simulink model "trajec_motion"  (R2016b)
settings: Solver=VariableStepAuto  StartTime=0.0  StopTime=10  RelTol=1e-3
undefined symbols (not defined in the file): X, Y, Z
libraries: sm_lib x12, nesl_utility x9, simulink x6
settings Model: Creator=macbookpro  LastModifiedBy=macbookpro
settings SimscapeCC: SimscapeLogType=all  SimscapeLogDataHistory=10000

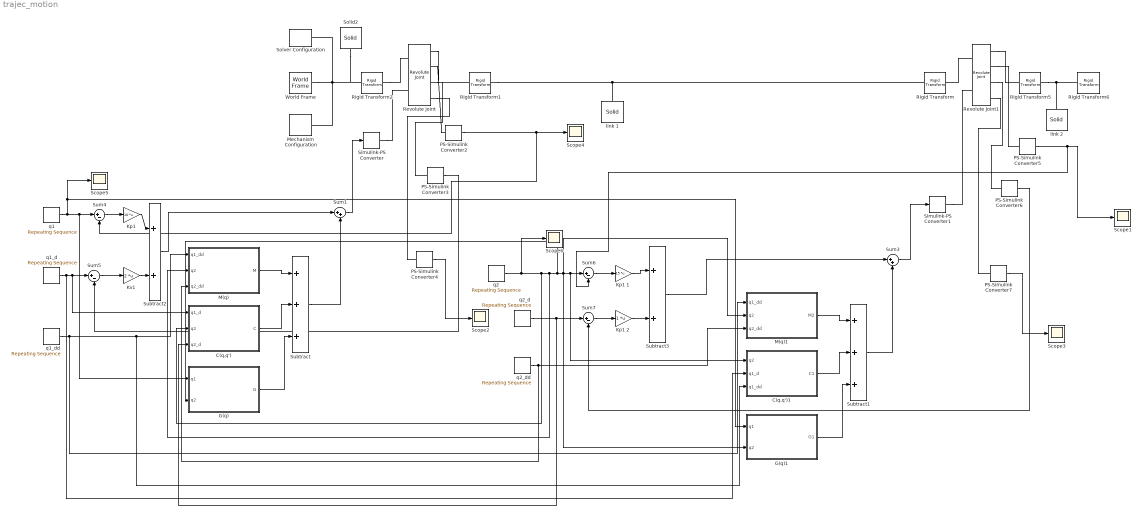
== system trajec_motion ==
  C(q,q') : MATLAB Function  TreatAsAtomicUnit=on
  C(q,q')1 : MATLAB Function  TreatAsAtomicUnit=on
  G(q) : MATLAB Function  TreatAsAtomicUnit=on
  G(q)1 : MATLAB Function  TreatAsAtomicUnit=on
  "Kp1 " : Gain  Gain=10  Multiplication=Matrix(K*u) (u vector)
  Kp1 1 : Gain  Gain=15  Multiplication=Matrix(K*u) (u vector)
  Kp1 2 : Gain  Multiplication=Matrix(K*u) (u vector)
  Kv1 : Gain  Gain=2  Multiplication=Matrix(K*u) (u vector)
  M(q) : MATLAB Function  TreatAsAtomicUnit=on
  M(q)1 : MATLAB Function  TreatAsAtomicUnit=on
  Mechanism Configuration : sm_lib/Utilities/Mechanism Configuration  UniformGravity=Constant  GravityVector=[0 0 -9.80665]  GravityUnits=m/s^2  LinearizationDelta=0.001
  PS-Simulink Converter2 : nesl_utility/PS-Simulink Converter  PhysicalDomain=network_engine_domain  SubClassName=ps_output  LeftPortType=input  RightPortType=output  PseudoPeriodic=off  Frequencies=[]  Unit=rad  AffineConversion=off
  PS-Simulink Converter3 : nesl_utility/PS-Simulink Converter  PhysicalDomain=network_engine_domain  SubClassName=ps_output  LeftPortType=input  RightPortType=output  PseudoPeriodic=off  Frequencies=[]  Unit=rad/s  AffineConversion=off
  PS-Simulink Converter4 : nesl_utility/PS-Simulink Converter  PhysicalDomain=network_engine_domain  SubClassName=ps_output  LeftPortType=input  RightPortType=output  PseudoPeriodic=off  Frequencies=[]  Unit=1  AffineConversion=off
  PS-Simulink Converter5 : nesl_utility/PS-Simulink Converter  PhysicalDomain=network_engine_domain  SubClassName=ps_output  LeftPortType=input  RightPortType=output  PseudoPeriodic=off  Frequencies=[]  Unit=rad  AffineConversion=off
  PS-Simulink Converter6 : nesl_utility/PS-Simulink Converter  PhysicalDomain=network_engine_domain  SubClassName=ps_output  LeftPortType=input  RightPortType=output  PseudoPeriodic=off  Frequencies=[]  Unit=rad/s  AffineConversion=off
  PS-Simulink Converter7 : nesl_utility/PS-Simulink Converter  PhysicalDomain=network_engine_domain  SubClassName=ps_output  LeftPortType=input  RightPortType=output  PseudoPeriodic=off  Frequencies=[]  Unit=1  AffineConversion=off
  Revolute Joint : sm_lib/Joints/Revolute Joint  SenseConstraintForce=off  SenseConstraintForceX=off  SenseConstraintForceY=off  SenseConstraintForceZ=off  SenseConstraintTorque=off  SenseConstraintTorqueX=off  SenseConstraintTorqueY=off  SenseConstraintTorqueZ=off  SenseTotalForce=off  SenseTotalForceX=off  SenseTotalForceY=off  SenseTotalForceZ=off  SenseTotalTorque=off  SenseTotalTorqueX=off  SenseTotalTorqueY=off  SenseTotalTorqueZ=off  CompositeWrenchDir=FollowerOnBase  CompositeWrenchFrame=BaseFrame  EquilibriumPosition=0  EquilibriumPositionUnits=rad  SpringStiffness=1  SpringStiffnessUnits=N*m/rad  DampingCoefficient=0.01  DampingCoefficientUnits=N*m/(rad/s)  TorqueActuationMode=InputTorque  MotionActuationMode=ComputedMotion  SensePosition=on  SenseVelocity=on  SenseAcceleration=on  SenseTorqueForce=off  PositionTargetSpecify=off  PositionTargetPriority=High  PositionTargetValue=30  PositionTargetValueUnits=deg  VelocityTargetSpecify=off  VelocityTargetPriority=High  VelocityTargetValue=0  VelocityTargetValueUnits=deg/s
  Revolute Joint1 : sm_lib/Joints/Revolute Joint  SenseConstraintForce=off  SenseConstraintForceX=off  SenseConstraintForceY=off  SenseConstraintForceZ=off  SenseConstraintTorque=off  SenseConstraintTorqueX=off  SenseConstraintTorqueY=off  SenseConstraintTorqueZ=off  SenseTotalForce=off  SenseTotalForceX=off  SenseTotalForceY=off  SenseTotalForceZ=off  SenseTotalTorque=off  SenseTotalTorqueX=off  SenseTotalTorqueY=off  SenseTotalTorqueZ=off  CompositeWrenchDir=FollowerOnBase  CompositeWrenchFrame=BaseFrame  EquilibriumPosition=0  EquilibriumPositionUnits=rad  SpringStiffness=1  SpringStiffnessUnits=N*m/rad  DampingCoefficient=0.01  DampingCoefficientUnits=N*m/(rad/s)  TorqueActuationMode=InputTorque  MotionActuationMode=ComputedMotion  SensePosition=on  SenseVelocity=on  SenseAcceleration=on  SenseTorqueForce=off  PositionTargetSpecify=off  PositionTargetPriority=High  PositionTargetValue=30  PositionTargetValueUnits=deg  VelocityTargetSpecify=off  VelocityTargetPriority=High  VelocityTargetValue=0  VelocityTargetValueUnits=deg/s
  Rigid Transform : sm_lib/Frames and Transforms/Rigid Transform  TranslationMethod=StandardAxis  TranslationStandardOffset=0.41/2  TranslationLengthUnit=m  TranslationStandardAxis=+Z  TranslationCartesianOffset=[0 0 0]  TranslationROffset=0  TranslationROffsetUnits=m  TranslationZOffset=0  TranslationZOffsetUnits=m  TranslationThetaOffset=0  TranslationThetaOffsetUnits=deg  RotationMethod=StandardAxis  RotationAngleUnits=deg  RotationStandardAxis=+X  RotationAngle=90  RotationArbitraryAxis=[0 0 1]  FollAlignAxisA=+X  BaseAlignAxisA=+Y  FollAlignAxisB=+Y  BaseAlignAxisB=+Z  RotationSequenceAxes=FollowerAxes  RotationSequence=XYX  RotationSequenceAngles=[0 0 0]  RotationSequenceAnglesUnits=deg  RotationMatrix=[1 0 0; 0 1 0; 0 0 1]
  Rigid Transform1 : sm_lib/Frames and Transforms/Rigid Transform  TranslationMethod=StandardAxis  TranslationStandardOffset=0.41/2  TranslationLengthUnit=m  TranslationStandardAxis=-Z  TranslationCartesianOffset=[0 0 0]  TranslationROffset=0  TranslationROffsetUnits=m  TranslationZOffset=0  TranslationZOffsetUnits=m  TranslationThetaOffset=0  TranslationThetaOffsetUnits=deg  RotationMethod=StandardAxis  RotationAngleUnits=deg  RotationStandardAxis=+X  RotationAngle=90  RotationArbitraryAxis=[0 0 1]  FollAlignAxisA=+X  BaseAlignAxisA=+Y  FollAlignAxisB=+Y  BaseAlignAxisB=+Z  RotationSequenceAxes=FollowerAxes  RotationSequence=XYX  RotationSequenceAngles=[0 0 0]  RotationSequenceAnglesUnits=deg  RotationMatrix=[1 0 0; 0 1 0; 0 0 1]
  Rigid Transform2 : sm_lib/Frames and Transforms/Rigid Transform  TranslationMethod=None  TranslationStandardOffset=0.41/2  TranslationLengthUnit=m  TranslationStandardAxis=+Z  TranslationCartesianOffset=[0 0 0]  TranslationROffset=0  TranslationROffsetUnits=m  TranslationZOffset=0  TranslationZOffsetUnits=m  TranslationThetaOffset=0  TranslationThetaOffsetUnits=deg  RotationMethod=StandardAxis  RotationAngleUnits=deg  RotationStandardAxis=+X  RotationAngle=90  RotationArbitraryAxis=[0 0 1]  FollAlignAxisA=+X  BaseAlignAxisA=+Y  FollAlignAxisB=+Y  BaseAlignAxisB=+Z  RotationSequenceAxes=FollowerAxes  RotationSequence=XYX  RotationSequenceAngles=[0 0 0]  RotationSequenceAnglesUnits=deg  RotationMatrix=[1 0 0; 0 1 0; 0 0 1]
  Rigid Transform5 : sm_lib/Frames and Transforms/Rigid Transform  TranslationMethod=StandardAxis  TranslationStandardOffset=0.39/2  TranslationLengthUnit=m  TranslationStandardAxis=-Z  TranslationCartesianOffset=[0 0 0]  TranslationROffset=0  TranslationROffsetUnits=m  TranslationZOffset=0  TranslationZOffsetUnits=m  TranslationThetaOffset=0  TranslationThetaOffsetUnits=deg  RotationMethod=StandardAxis  RotationAngleUnits=deg  RotationStandardAxis=+X  RotationAngle=90  RotationArbitraryAxis=[0 0 1]  FollAlignAxisA=+X  BaseAlignAxisA=+Y  FollAlignAxisB=+Y  BaseAlignAxisB=+Z  RotationSequenceAxes=FollowerAxes  RotationSequence=XYX  RotationSequenceAngles=[0 0 0]  RotationSequenceAnglesUnits=deg  RotationMatrix=[1 0 0; 0 1 0; 0 0 1]
  Rigid Transform6 : sm_lib/Frames and Transforms/Rigid Transform  TranslationMethod=StandardAxis  TranslationStandardOffset=0.39/2  TranslationLengthUnit=m  TranslationStandardAxis=+Z  TranslationCartesianOffset=[0 0 0]  TranslationROffset=0  TranslationROffsetUnits=m  TranslationZOffset=0  TranslationZOffsetUnits=m  TranslationThetaOffset=0  TranslationThetaOffsetUnits=deg  RotationMethod=StandardAxis  RotationAngleUnits=deg  RotationStandardAxis=+X  RotationAngle=90  RotationArbitraryAxis=[0 0 1]  FollAlignAxisA=+X  BaseAlignAxisA=+Y  FollAlignAxisB=+Y  BaseAlignAxisB=+Z  RotationSequenceAxes=FollowerAxes  RotationSequence=XYX  RotationSequenceAngles=[0 0 0]  RotationSequenceAnglesUnits=deg  RotationMatrix=[1 0 0; 0 1 0; 0 0 1]
  Scope{1..6} (6 alike) : Scope
  Simulink-PS Converter : nesl_utility/Simulink-PS Converter  PhysicalDomain=network_engine_domain  SubClassName=ps_input  LeftPortType=input  RightPortType=output  PseudoPeriodic=off  Frequencies=[]  NoiseDistribution=none  NoiseParameters=[]  Unit=N*m  AffineConversion=off  InputFiltering=on  SimscapeFilterOrder=2  InputFilterTimeConstant=0.01  UdotUserProvided=1
  Simulink-PS Converter1 : nesl_utility/Simulink-PS Converter  PhysicalDomain=network_engine_domain  SubClassName=ps_input  LeftPortType=input  RightPortType=output  PseudoPeriodic=off  Frequencies=[]  NoiseDistribution=none  NoiseParameters=[]  Unit=N*m  AffineConversion=off  InputFiltering=on  SimscapeFilterOrder=2  InputFilterTimeConstant=0.01  UdotUserProvided=1
  Solid2 : sm_lib/Body Elements/Solid  InertiaType=CalculateFromGeometry  Mass=1  MassUnits=kg  CenterOfMass=[0 0 0]  CenterOfMassUnits=m  MomentsOfInertia=[1 1 1]  MomentsOfInertiaUnits=kg*m^2  ProductsOfInertia=[1 1 1]  ProductsOfInertiaUnits=kg*m^2  DensityBased=on  Density=4000  DensityUnits=kg/m^3  DoExposeReferenceFrame=on  SerializedFrames=<Frames/>  GraphicType=FromGeometry  MarkerShape=Sphere  MarkerSize=10  GraphicVisPropType=SimpleVisualProperties  GraphicDiffuseColor=[0.5 0.5 0.5]  GraphicSpecularColor=[0.5 0.5 0.5 1.0]  GraphicAmbientColor=[0.15 0.15 0.15 1.0]  GraphicEmissiveColor=[0.0 0.0 0.0 1.0]  GraphicShininess=75  GraphicOpacity=1.0  GeometryShape=Brick  RectangleSize=[1 1]  RectangleSizeUnits=m  BrickDimensions=[1.5 0.5 0.05]  BrickDimensionUnits=m  CylinderRadius=0.02  CylinderRadiusUnits=m  CylinderLength=0.41  CylinderLengthUnits=m  SphereRadius=1  SphereRadiusUnits=m  EllipsoidRadii=[1 1 1]  EllipsoidRadiiUnits=m  ExtrusionCrossSection=[1 1; -1 1; -1 -1; 1 -1]  ExtrusionCrossSectionUnits=m  ExtrusionLength=1  ExtrusionLengthUnits=m  PolygonNumSides=3  PolygonOuterRadius=1  PolygonOuterRadiusUnits=m  ExtGeomFileType=STEP  ExtGeomFileUnits=m  RevolutionCrossSection=[1 1; 1 -1; 2 -1; 2 1]  RevolutionCrossSectionUnits=m  RevolutionExtent=Full  RevolutionAngle=180  RevolutionAngleUnits=deg
  Solver Configuration : nesl_utility/Solver Configuration  PhysicalDomain=network_engine_domain  SubClassName=solver  LeftPortType=input  RightPortType=generic  Accelerate=off  Tones=[]  Harmonics=[]  SimulateNoise=off  Profile=off  UseLocalSampling=off  EnableSwitchedLinearOptims=on  FrequencyDomain=off  UseCCode=off  RelTol=0.001  AbsTol=1e-06  MinStep=1e-09  ToWorkspace=off  RevertToSquareIcSolve=off  NumHomotopyIterations=100  PhasorMode=off  PhasorModeNumHarmonics=1  OverrideAbsTol=off  DoDC=off  ResidualTolerance=1e-09  UseLocalSolver=off  LocalSolverChoice=NE_BACKWARD_EULER_ADVANCER  LocalSolverSampleTime=0.001  DoFixedCost=off  MaxNonlinIter=3  MaxModeIter=2  LinearAlgebra=Sparse  DelaysMemoryBudget=1024  AutomaticFiltering=on  FilteringTimeConstant=0.001
  Subtract : Sum  Inputs=+++
  Subtract1 : Sum  Inputs=+++
  Subtract2 : Sum
  Subtract3 : Sum
  Sum1 : Sum  Inputs=|++
  Sum3 : Sum  Inputs=|++
  Sum{4..7} (4 alike) : Sum  Inputs=|+-
  World Frame : sm_lib/Frames and Transforms/World Frame
  link 1 : sm_lib/Body Elements/Solid  InertiaType=CalculateFromGeometry  Mass=1  MassUnits=kg  CenterOfMass=[0 0 0]  CenterOfMassUnits=m  MomentsOfInertia=[1 1 1]  MomentsOfInertiaUnits=kg*m^2  ProductsOfInertia=[1 1 1]  ProductsOfInertiaUnits=kg*m^2  DensityBased=on  Density=4542  DensityUnits=kg/m^3  DoExposeReferenceFrame=on  SerializedFrames=<Frames/>  GraphicType=FromGeometry  MarkerShape=Sphere  MarkerSize=10  GraphicVisPropType=SimpleVisualProperties  GraphicDiffuseColor=[0.5 0.5 0.5]  GraphicSpecularColor=[0.5 0.5 0.5 1.0]  GraphicAmbientColor=[0.15 0.15 0.15 1.0]  GraphicEmissiveColor=[0.0 0.0 0.0 1.0]  GraphicShininess=75  GraphicOpacity=1.0  GeometryShape=Cylinder  RectangleSize=[1 1]  RectangleSizeUnits=m  BrickDimensions=[1 1 1]  BrickDimensionUnits=m  CylinderRadius=0.02  CylinderRadiusUnits=m  CylinderLength=0.41  CylinderLengthUnits=m  SphereRadius=1  SphereRadiusUnits=m  EllipsoidRadii=[1 1 1]  EllipsoidRadiiUnits=m  ExtrusionCrossSection=[1 1; -1 1; -1 -1; 1 -1]  ExtrusionCrossSectionUnits=m  ExtrusionLength=1  ExtrusionLengthUnits=m  PolygonNumSides=3  PolygonOuterRadius=1  PolygonOuterRadiusUnits=m  ExtGeomFileType=STEP  ExtGeomFileUnits=m  RevolutionCrossSection=[1 1; 1 -1; 2 -1; 2 1]  RevolutionCrossSectionUnits=m  RevolutionExtent=Full  RevolutionAngle=180  RevolutionAngleUnits=deg
  link 2 : sm_lib/Body Elements/Solid  InertiaType=CalculateFromGeometry  Mass=1  MassUnits=kg  CenterOfMass=[0 0 0]  CenterOfMassUnits=m  MomentsOfInertia=[1 1 1]  MomentsOfInertiaUnits=kg*m^2  ProductsOfInertia=[1 1 1]  ProductsOfInertiaUnits=kg*m^2  DensityBased=on  Density=5162  DensityUnits=kg/m^3  DoExposeReferenceFrame=on  SerializedFrames=<Frames/>  GraphicType=FromGeometry  MarkerShape=Sphere  MarkerSize=10  GraphicVisPropType=SimpleVisualProperties  GraphicDiffuseColor=[0.5 0.5 0.5]  GraphicSpecularColor=[0.5 0.5 0.5 1.0]  GraphicAmbientColor=[0.15 0.15 0.15 1.0]  GraphicEmissiveColor=[0.0 0.0 0.0 1.0]  GraphicShininess=75  GraphicOpacity=1.0  GeometryShape=Cylinder  RectangleSize=[1 1]  RectangleSizeUnits=m  BrickDimensions=[1 1 1]  BrickDimensionUnits=m  CylinderRadius=0.02  CylinderRadiusUnits=m  CylinderLength=0.39  CylinderLengthUnits=m  SphereRadius=1  SphereRadiusUnits=m  EllipsoidRadii=[1 1 1]  EllipsoidRadiiUnits=m  ExtrusionCrossSection=[1 1; -1 1; -1 -1; 1 -1]  ExtrusionCrossSectionUnits=m  ExtrusionLength=1  ExtrusionLengthUnits=m  PolygonNumSides=3  PolygonOuterRadius=1  PolygonOuterRadiusUnits=m  ExtGeomFileType=STEP  ExtGeomFileUnits=m  RevolutionCrossSection=[1 1; 1 -1; 2 -1; 2 1]  RevolutionCrossSectionUnits=m  RevolutionExtent=Full  RevolutionAngle=180  RevolutionAngleUnits=deg
  q1 : simulink/Sources/Repeating Sequence  rep_seq_t=tt  rep_seq_y=q1
  q1_d : simulink/Sources/Repeating Sequence  rep_seq_t=tt  rep_seq_y=q1_d
  q1_dd : simulink/Sources/Repeating Sequence  rep_seq_t=tt  rep_seq_y=q1_dd
  q2 : simulink/Sources/Repeating Sequence  rep_seq_t=tt  rep_seq_y=q2
  q2_d : simulink/Sources/Repeating Sequence  rep_seq_t=tt  rep_seq_y=q2_d
  q2_dd : simulink/Sources/Repeating Sequence  rep_seq_t=tt  rep_seq_y=q2_dd
  wires:
  Sum1/1 -> Simulink-PS Converter/1
  Sum3/1 -> Simulink-PS Converter1/1
  Subtract2/1 -> Sum1/1
  q1_d/1 -> C(q,q')1/2(q1_d), C(q,q')/1(q1_d), Sum5/1
  M(q)/1(M) -> Subtract/1
  C(q,q')/1(C) -> Subtract/2
  G(q)/1(G) -> Subtract/3
  Subtract/1 -> Sum1/2
  PS-Simulink Converter3/1 -> Sum5/2
  PS-Simulink Converter4/1 -> Scope2/1
  Subtract3/1 -> Sum3/1
  M(q)1/1(M2) -> Subtract1/1
  C(q,q')1/1(C1) -> Subtract1/2
  G(q)1/1(G1) -> Subtract1/3
  Subtract1/1 -> Sum3/2
  PS-Simulink Converter6/1 -> Sum7/2
  PS-Simulink Converter7/1 -> Scope3/1
  q1/1 -> Scope5/1, G(q)1/1(q1), G(q)/1(q1), Sum4/1
  Sum4/1 -> "Kp1 "/1
  Sum5/1 -> Kv1/1
  "Kp1 "/1 -> Subtract2/1
  Kv1/1 -> Subtract2/2
  q1_dd/1 -> M(q)1/1(q1_dd), C(q,q')1/3(q1_dd), M(q)/1(q1_dd)
  q2/1 -> Scope6/1, C(q,q')/2(q2), M(q)/2(q2), G(q)/2(q2), G(q)1/2(q2), M(q)1/2(q2), C(q,q')1/1(q2), Sum6/1
  Sum6/1 -> Kp1 1/1
  q2_d/1 -> C(q,q')/3(q2_d), Sum7/1
  Sum7/1 -> Kp1 2/1
  Kp1 2/1 -> Subtract3/2
  Kp1 1/1 -> Subtract3/1
  q2_dd/1 -> M(q)/3(q2_dd), M(q)1/3(q2_dd)
  PS-Simulink Converter2/1 -> Scope4/1, Sum4/2
  PS-Simulink Converter5/1 -> Sum6/2, Scope1/1
  connections:
  World Frame/RConn1 -- Solid2/RConn1 -- Rigid Transform2/LConn1 -- Solver Configuration/RConn1 -- Mechanism Configuration/RConn1
  link 1/RConn1 -- Rigid Transform/LConn1 -- Rigid Transform1/LConn1
  Revolute Joint/RConn1 -- Rigid Transform1/RConn1
  Rigid Transform2/RConn1 -- Revolute Joint/LConn1
  Revolute Joint1/LConn1 -- Rigid Transform/RConn1
  link 2/RConn1 -- Rigid Transform6/LConn1 -- Rigid Transform5/LConn1
  Revolute Joint1/RConn1 -- Rigid Transform5/RConn1
  Simulink-PS Converter/RConn1 -- Revolute Joint/LConn2
  Simulink-PS Converter1/RConn1 -- Revolute Joint1/LConn2
  Revolute Joint/RConn2 -- PS-Simulink Converter2/LConn1
  Revolute Joint/RConn3 -- PS-Simulink Converter3/LConn1
  Revolute Joint/RConn4 -- PS-Simulink Converter4/LConn1
  Revolute Joint1/RConn2 -- PS-Simulink Converter5/LConn1
  Revolute Joint1/RConn3 -- PS-Simulink Converter6/LConn1
  Revolute Joint1/RConn4 -- PS-Simulink Converter7/LConn1

== matlab function trajec_motion/G(q) ==
  data: q1 input; G output; q2 input
function G = fcn(q1,q2)
l1=0.41;% m
l2=0.39; % m
m1=2.34;%kg
m2=2.53;%kg
J1=0.76;%kgm^2
J2=0.69;%kgm^2
g=9.81;%kg/m^2
G=1/2*m1*g*l1*cos(q1)+1/2*m2*g*l2*cos((q1+q2))+m2*g*l1*cos(q1);
end

== matlab function trajec_motion/M(q) ==
  data: M output; q1_dd input; q2 input; q2_dd input
function M = fcn(q1_dd,q2,q2_dd)
l1=0.41;% m
l2=0.39; % m
m1=2.34;%kg
m2=2.53;%kg
J1=0.76;%kgm^2
J2=0.69;%kgm^2
M=(0.76+m2*l1^2+m2*l1*l2*cos(q2)+J2)*q1_dd+(J2+1/2*m2*l1*l2*cos(q2))*q2_dd;
end

== matlab function trajec_motion/C(q,q') ==
  data: C output; q1_d input; q2 input; q2_d input
function C = fcn(q1_d,q2,q2_d)
l1=0.41;% m
l2=0.39; % m
m1=2.34;%kg
m2=2.53;%kg
J1=0.76;%kgm^2
J2=0.69;%kgm^2
C=(-1/2*m2*l1*l2*sin(q2)*q2_d)*q1_d+(-1/2*m2*l1*l2*sin((q1_d+q2_d)))*q2_d;
end

== matlab function trajec_motion/C(q,q')1 ==
  data: q2 input; C1 output; q1_d input; q1_dd input
function C1 = fcn(q2,q1_d,q1_dd)
l1=0.41;% m
l2=0.39; % m
m1=2.34;%kg
m2=2.53;%kg
J1=0.76;%kgm^2
J2=0.69;%kgm^2
C1=1/2*m2*l1*l2*sin(q2)*q1_d*q1_dd;
end

== matlab function trajec_motion/G(q)1 ==
  data: q1 input; G1 output; q2 input
function G1 = fcn(q1,q2)
l1=0.41;% m
l2=0.39; % m
m1=2.34;%kg
m2=2.53;%kg
J1=0.76;%kgm^2
J2=0.69;%kgm^2
g=9.81;%kg/m^2
G1=1/2*m2*g*l2*cos((q1+q2));
end

== matlab function trajec_motion/M(q)1 ==
  data: q1_dd input; M2 output; q2 input; q2_dd input
function M2 = fcn(q1_dd,q2,q2_dd)

l1=0.41;% m
l2=0.39; % m
m1=2.34;%kg
m2=2.53;%kg
J1=0.76;%kgm^2
J2=0.69;%kgm^2
M2=(J1+1/2*m2*l1*l2*cos(q2))*q1_dd+J2*q2_dd;
end
